simulink model "practice_2"  (R2020a)
settings: Solver=VariableStepAuto  StartTime=0.0  StopTime=10  RelTol=1e-3
settings Model: Creator=Riyansh  LastModifiedBy=Riyansh

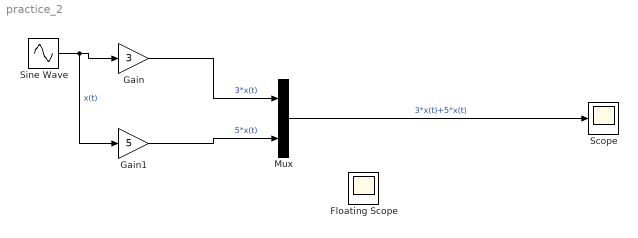
== system practice_2 ==
  Floating Scope : Scope
      settings: Floating=on
  Gain : Gain  Gain=3
  Gain1 : Gain  Gain=5
  Mux : Mux  Inputs=2
  Scope : Scope
  Sine Wave : Sin  SampleTime=0
  wires:
  Sine Wave/1 -> Gain1/1, Gain/1  "x(t)"
  Gain/1 -> Mux/1  "3*x(t)"
  Gain1/1 -> Mux/2  "5*x(t)"
  Mux/1 -> Scope/1  "3*x(t)+5*x(t)"
